simulink subsystem "ControladorBA"  (R2023b)
settings: Solver=VariableStepAuto  StartTime=0.0  StopTime=10.0  RelTol=1e-3
settings Model: Creator=manu_  LastModifiedBy=manu_

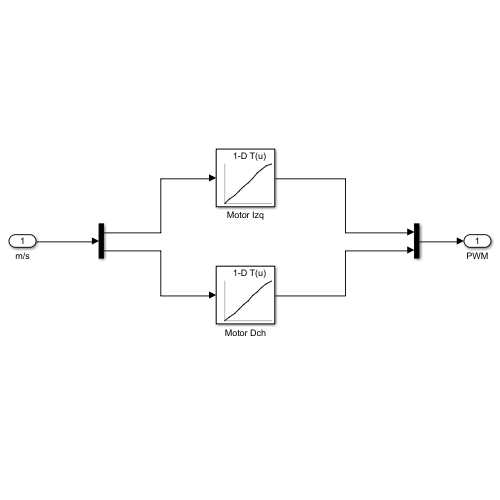
[thumbnail: Simulink's stored preview of the top-level diagram]
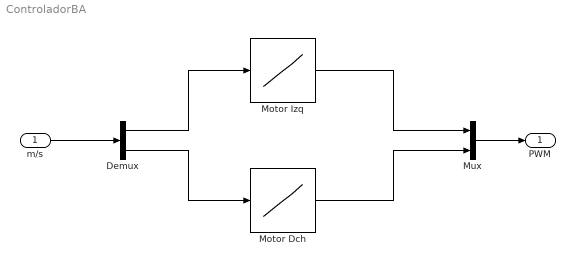
== system ControladorBA ==
  m/s : Inport
  Demux : Demux  Outputs=2
  "Motor Dch " : Lookup_n-D  NumberOfTableDimensions=1  BreakpointsForDimension1=[-255 -200 -150 -100 -50 0 50 100 150 200 255]  Table=[-0.4536 -0.3654 -0.2772 -0.1819 -0.0756 0 0.126 0.2142 0.315 0.4032 0.4662]  InternalRulePriority=Speed  RndMeth=Simplest
  "Motor Izq " : Lookup_n-D  NumberOfTableDimensions=1  BreakpointsForDimension1=[-255 -200 -150 -100 -50 0 50 100 150 200 255]  Table=[-0.4788 -0.378 -0.2898 -0.189 -0.0756 0 0.1134 0.2268 0.315 0.4032 0.4536]  InternalRulePriority=Speed  RndMeth=Simplest
  Mux : Mux  Inputs=2
  PWM : Outport
  wires:
  Demux/1 -> "Motor Izq "/1
  m/s/1 -> Demux/1
  Mux/1 -> PWM/1
  Demux/2 -> "Motor Dch "/1
  "Motor Izq "/1 -> Mux/1
  "Motor Dch "/1 -> Mux/2
